simulink model "modulation_cosim"  (Simulink 6.3)
settings: Solver=FixedStepDiscrete  StartTime=0.0  StopTime=10.0  RelTol=1e-3
undefined symbols (not defined in the file): image, port_label
libraries: aldec_ahdl x5
settings Model: LastModifiedBy=arekg
settings DataIOCC: SignalLoggingName=sigsOut
settings OptimizationCC: InlineInvariantSignals=on
settings DebuggingCC: SolverPrmCheckMsg=none
settings HardwareCC: TargetUnknown=on
settings GRTTargetCC: ModelReferenceCompliant=off  MatFileLogging=off

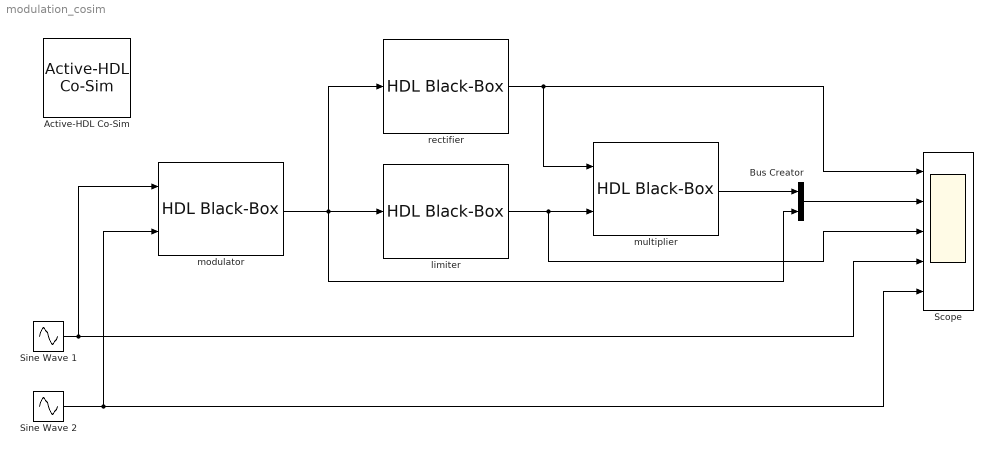
== system modulation_cosim ==
  Active-HDL Co-Sim : aldec_ahdl/Active-HDL Co-Sim  hdl_period=1/20  hdl_tscale=sec  sys_period=1/20  sys_tscale=As In Simulator  wav_fn=mlab_cosim  wav_settings=[0,0,0,0]  dbg=off  auto_start=off  gen_tb=off  batch_sim=off  tb_fn=mlab_post_tb.log  metavalue_map=[0,0]  sim_resolution=[1,0,0]  active_page=2
  Bus Creator : BusCreator  Inputs=2
  Scope : Scope  NumInputPorts=5
      settings: YMin=-1~-40~-2~-1~-1.5  YMax=40~40~2~40~1.5
  Sine Wave 1 : Sin  Amplitude=18  Bias=20  Frequency=0.5*pi  Phase=pi/1.3  SampleTime=1/20
  Sine Wave 2 : Sin  Amplitude=0.9  Frequency=pi/0.4  Phase=pi  SampleTime=1/20
  limiter : aldec_ahdl/HDL Black-Box  module_m=signum  ports_cfg={In1,0,31,24,24,1,0,0,0,0,0,0}{Out1,1,2,0,0,1,0,0,0,0,0,0}  hdl_src=c:\My_Designs\Samples_72\simulink_example\Modulation\src\sign.vhd  block_mask=image(imread('HDLBlackBox.jpg'),'center'); disp('signum');port_label('input', 1, 'In1'); port_label('output', 1, 'Out1');  inp=[1,0,31,24]  out=[1,0,2,0]  sampling=[0,1]  active_page=0  param_val=0  port_in_val=0  port_out_val=0  clk_val=0  ce_val=0  config=0
  modulator : aldec_ahdl/HDL Black-Box  module_m=mult  ports_cfg={Sin_wav1,0,16,9,9,1,0,0,0,0,0,0}{Sin_wav2,0,16,15,15,1,0,0,0,0,0,0}{Out1,1,31,24,24,1,0,0,0,0,0,0}  hdl_src=c:\My_Designs\Samples_72\simulink_example\Modulation\src\mult.vhd  block_mask=image(imread('HDLBlackBox.jpg'),'center'); disp('mult');port_label('input', 1, 'Sin_wav1'); port_label('input', 2, 'Sin_wav2'); port_label('output', 1, 'Out1');  inp=[2,0,16,9,0,16,15]  out=[1,0,31,24]  sampling=[0,1]  active_page=0  param_val=0  port_in_val=0  port_out_val=0  clk_val=0  ce_val=0  config=0
  multiplier : aldec_ahdl/HDL Black-Box  module_m=mult1  ports_cfg={I_abs,0,31,24,24,1,0,0,0,0,0,0}{I_sig,0,2,0,0,1,0,0,0,0,0,0}{Out1,1,31,24,24,1,0,0,0,0,0,0}  hdl_src=c:\My_Designs\Samples_72\simulink_example\Modulation\src\mult1.vhd  block_mask=image(imread('HDLBlackBox.jpg'),'center'); disp('mult1');port_label('input', 1, 'I_abs'); port_label('input', 2, 'I_sig'); port_label('output', 1, 'Out1');  inp=[2,0,31,24,0,2,0]  out=[1,0,31,24]  sampling=[0,1]  active_page=0  param_val=0  port_in_val=0  port_out_val=0  clk_val=0  ce_val=0  config=0
  rectifier : aldec_ahdl/HDL Black-Box  module_m=m_abs  ports_cfg={In1,0,31,24,24,1,0,0,0,0,0,0}{Out1,1,31,24,24,1,0,0,0,0,0,0}  hdl_src=c:\My_Designs\Samples_72\simulink_example\Modulation\src\abs.vhd  block_mask=image(imread('HDLBlackBox.jpg'),'center'); disp('m_abs');port_label('input', 1, 'In1'); port_label('output', 1, 'Out1');  inp=[1,0,31,24]  out=[1,0,31,24]  sampling=[0,1]  active_page=0  param_val=0  port_in_val=0  port_out_val=0  clk_val=0  ce_val=0  config=0
  wires:
  rectifier/1 -> Scope/1, multiplier/1
  Sine Wave 1/1 -> Scope/4, modulator/1
  Sine Wave 2/1 -> Scope/5, modulator/2
  modulator/1 -> Bus Creator/2, limiter/1, rectifier/1
  limiter/1 -> Scope/3, multiplier/2
  multiplier/1 -> Bus Creator/1
  Bus Creator/1 -> Scope/2
